simulink model "freerunsom"  (Simulink 4.00)
settings: Solver=ode45  SolverMode=SingleTasking  StartTime=0.0  StopTime=250  RelTol=1e-3  AbsTol=1e-3
settings Model: LastModifiedBy=abonyij  SaveTime=off  SaveOutput=off  LimitDataPoints=off  RTWTemplateMakefile=grt_vc.tmf  ExtModeTrigMode=oneshot  ExtModeArmWhenConnect=off  BlockReductionOpt=off

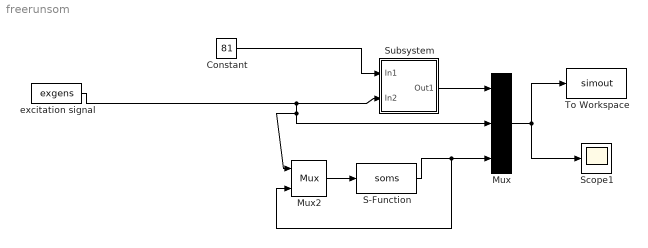
== system freerunsom ==
  Constant : Constant  Value=81
  Mux : Mux  Inputs=3
      settings: DisplayOption=none
  Mux2 : Mux  Inputs=2
      settings: DisplayOption=none
  S-Function : S-Function  FunctionName=soms  PortCounts=[]  SFunctionModules=''
  Scope1 : Scope
      settings: TickLabels=on  TimeRange=auto  YMin=6  YMax=12  SaveName=pi  DataFormat=Array  LimitDataPoints=on  MaxDataPoints=5000  SampleInput=on
  Subsystem : Subsystem
      settings: RTWFcnNameOpts=Auto  RTWFileNameOpts=Auto
  To Workspace : ToWorkspace  VariableName=simout  SampleTime=0.2  SaveFormat=Array
  excitation signal : S-Function  FunctionName=exgens  PortCounts=[]  SFunctionModules=''
  wires:
  Mux/1 -> Scope1/1, To Workspace/1
  Constant/1 -> Subsystem/1(In1)
  Subsystem/1(Out1) -> Mux/1
  Mux2/1 -> S-Function/1
  S-Function/1 -> Mux/3, Mux2/2
  excitation signal/1 -> Subsystem/2(In2), Mux/2, Mux2/1

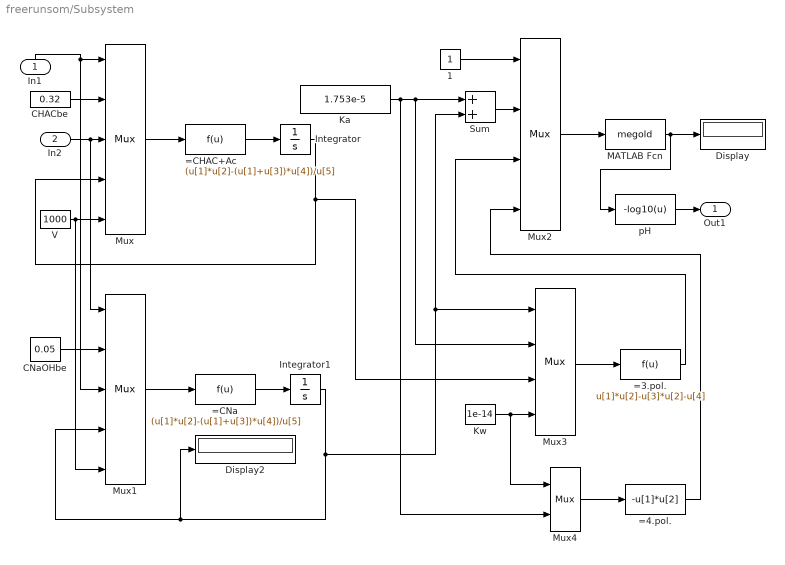
== system freerunsom/Subsystem ==
  In1 : Inport  Orientation=up  Port=1
  In2 : Inport  Port=2
  1 : Constant  Value=1
  =3.pol. : Fcn  Expr=u[1]*u[2]-u[3]*u[2]-u[4]
  =4.pol. : Fcn  Expr=-u[1]*u[2]
  =CHAC+Ac : Fcn  Expr=(u[1]*u[2]-(u[1]+u[3])*u[4])/u[5]
  =CNa : Fcn  Expr=(u[1]*u[2]-(u[1]+u[3])*u[4])/u[5]
  CHACbe : Constant  Value=0.32
  CNaOHbe : Constant  Value=0.05
  Display : Display
      settings: Format=short
  Display2 : Display
      settings: Format=short
  Integrator : Integrator  ExternalReset=none  InitialConditionSource=internal  InitialCondition=0.0435  LimitOutput=off  UpperSaturationLimit=inf  LowerSaturationLimit=-inf  ShowSaturationPort=off  ShowStatePort=off  AbsoluteTolerance=auto
  Integrator1 : Integrator  ExternalReset=none  InitialConditionSource=internal  InitialCondition=0.0432  LimitOutput=off  UpperSaturationLimit=inf  LowerSaturationLimit=-inf  ShowSaturationPort=off  ShowStatePort=off  AbsoluteTolerance=auto
  Ka : Constant  Value=1.753e-5
  Kw : Constant  Value=1e-14
  MATLAB Fcn : MATLABFcn  MATLABFcn=megold  OutputDimensions=1  OutputSignalType=auto  Output1D=on
  Mux : Mux  Inputs=5
      settings: DisplayOption=none
  Mux1 : Mux  Inputs=5
      settings: DisplayOption=none
  Mux2 : Mux  Inputs=4
      settings: DisplayOption=none
  Mux3 : Mux  Inputs=4
      settings: DisplayOption=none
  Mux4 : Mux  Inputs=2
      settings: DisplayOption=none
  Sum : Sum  Inputs=++  SaturateOnIntegerOverflow=on
  V : Constant  Value=1000
  pH : Fcn  Expr=-log10(u)
  Out1 : Outport  Port=1  InitialOutput=0
  wires:
  CHACbe/1 -> Mux/2
  Mux/1 -> =CHAC+Ac/1
  =CHAC+Ac/1 -> Integrator/1
  In2/1 -> Mux/3, Mux1/1
  CNaOHbe/1 -> Mux1/2
  In1/1 -> Mux/1, Mux1/3
  =CNa/1 -> Integrator1/1
  Mux1/1 -> =CNa/1
  V/1 -> Mux/5, Mux1/5
  1/1 -> Mux2/1
  Integrator1/1 -> Display2/1, Mux1/4, Sum/2, Mux3/1
  Mux3/1 -> =3.pol./1
  Integrator/1 -> Mux/4, Mux3/3
  Mux4/1 -> =4.pol./1
  Kw/1 -> Mux3/4, Mux4/1
  Ka/1 -> Sum/1, Mux3/2, Mux4/2
  Sum/1 -> Mux2/2
  =3.pol./1 -> Mux2/3
  =4.pol./1 -> Mux2/4
  Mux2/1 -> MATLAB Fcn/1
  MATLAB Fcn/1 -> Display/1, pH/1
  pH/1 -> Out1/1
